simulink model "doc_moqpskdemod_fb"  (R2014a)
settings: Solver=FixedStepDiscrete  StartTime=0.0  StopTime=6  RelTol=1e-3
libraries: commdigbbndpm3 x2
settings Model: Creator=The MathWorks Inc.
settings DataIOCC: SignalLoggingSaveFormat=ModelDataLogs
settings OptimizationCC: BlockReduction=off  ExpressionDepthLimit=2147483647  EfficientMapNaN2IntZero=off
settings DebuggingCC: UnderspecifiedInitializationDetection=Classic  FcnCallInpInsideContextMsg=UseLocalSettings  StateNameClashWarn=warning  StrictBusMsg=Warning
settings GRTTargetCC: CombineOutputUpdateFcns=off  GRTInterface=on

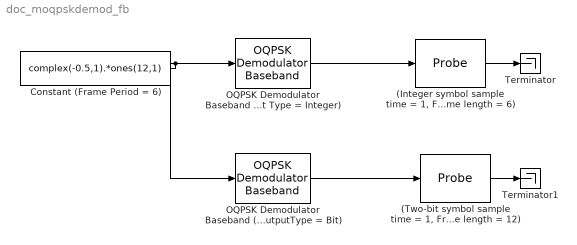
== system doc_moqpskdemod_fb ==
  "(Integer symbol sample time = 1, Frame length = 6)" : Probe  ProbeWidth=off  ProbeComplexSignal=off
  "(Two-bit symbol sample time = 1, Frame length = 12)" : Probe  ProbeWidth=off  ProbeComplexSignal=off
  Constant (Frame Period = 6) : Constant  Value=complex(-0.5,1).*ones(12,1)  VectorParams1D=off  SampleTime=1  FramePeriod=6
      settings: SamplingMode=Frame based
  OQPSK Demodulator Baseband (Output Type = Integer) : commdigbbndpm3/OQPSK Demodulator Baseband  OutType=Integer  Ph=0  RateOptions=Enforce single-rate processing  outDtype1=Inherit via internal rule  outDtype2=double  derotateFactorWordLen=16  roundingMode=Floor  overflowMode=Wrap
  OQPSK Demodulator Baseband (OutputType = Bit) : commdigbbndpm3/OQPSK Demodulator Baseband  OutType=Bit  Ph=0  RateOptions=Enforce single-rate processing  outDtype1=double  outDtype2=double  derotateFactorWordLen=16  roundingMode=Floor  overflowMode=Wrap
  Terminator : Terminator
  Terminator1 : Terminator
  wires:
  Constant (Frame Period = 6)/1 -> OQPSK Demodulator Baseband (OutputType = Bit)/1, OQPSK Demodulator Baseband (Output Type = Integer)/1
  OQPSK Demodulator Baseband (Output Type = Integer)/1 -> "(Integer symbol sample time = 1, Frame length = 6)"/1
  OQPSK Demodulator Baseband (OutputType = Bit)/1 -> "(Two-bit symbol sample time = 1, Frame length = 12)"/1
  "(Integer symbol sample time = 1, Frame length = 6)"/1 -> Terminator/1
  "(Two-bit symbol sample time = 1, Frame length = 12)"/1 -> Terminator1/1
